simulink model "task_2_sim"  (R2023a)
settings: Solver=VariableStepAuto  StartTime=0.0  StopTime=3  RelTol=1e-7
undefined symbols (not defined in the file): A, C, L1, x_0, x_h_0
settings Model: Creator=user  LastModifiedBy=user

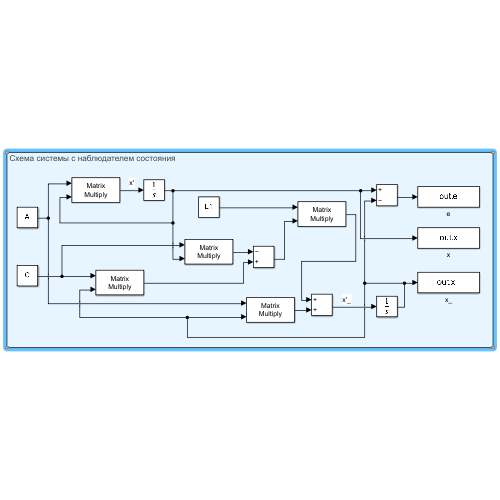
[thumbnail: Simulink's stored preview of the top-level diagram]
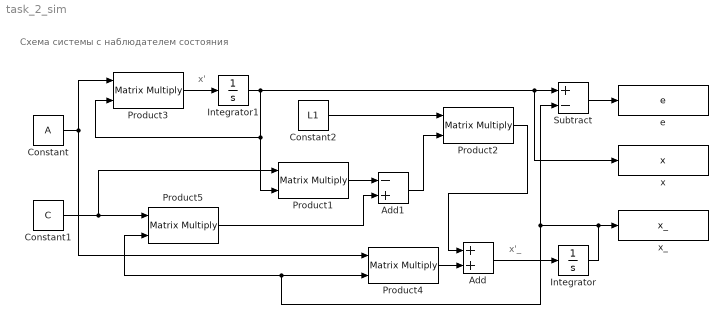
== system task_2_sim ==
  note: Схема системы с наблюдателем состояния
  note: x'
  note: x'_
  Add : Sum
  Add1 : Sum  Inputs=-+
  Constant : Constant  Value=A  VectorParams1D=off
  Constant1 : Constant  Value=C  VectorParams1D=off
  Constant2 : Constant  Value=L1  VectorParams1D=off
  Integrator : Integrator  InitialCondition=x_h_0
  Integrator1 : Integrator  InitialCondition=x_0
  Product{1..5} (5 alike) : Product  Multiplication=Matrix(*)
  Subtract : Sum  Inputs=+-
  e : ToWorkspace  VariableName=e  SaveFormat=Timeseries  SampleTime=-1
  x : ToWorkspace  VariableName=x  SaveFormat=Timeseries  SampleTime=-1
  x_ : ToWorkspace  VariableName=x_  SaveFormat=Timeseries  SampleTime=-1
  wires:
  Constant/1 -> Product4/1, Product3/1
  Product3/1 -> Integrator1/1
  Integrator1/1 -> Subtract/1, x/1, Product1/2, Product3/2
  Constant1/1 -> Product1/1, Product5/1
  Product1/1 -> Add1/1
  Add1/1 -> Product2/2
  Constant2/1 -> Product2/1
  Product2/1 -> Add/1
  Product4/1 -> Add/2
  Add/1 -> Integrator/1
  Integrator/1 -> x_/1, Product4/2, Product5/2, Subtract/2
  Product5/1 -> Add1/2
  Subtract/1 -> e/1
